simulink model "ex3"  (R2020a)
settings: Solver=VariableStepAuto  StartTime=0.0  StopTime=10.0  RelTol=1e-3
settings Model: Creator=EREN  LastModifiedBy=EREN

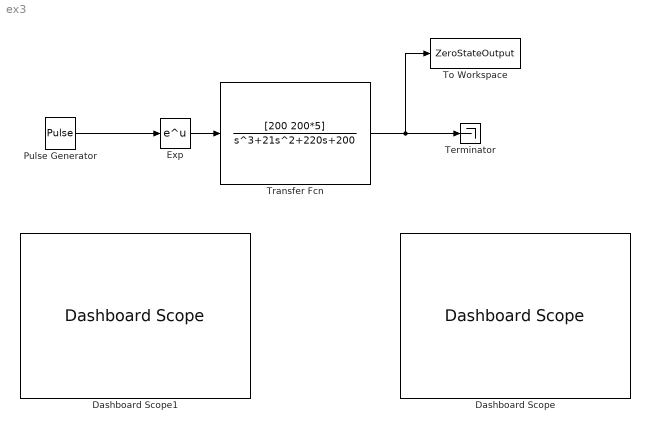
== system ex3 ==
  Dashboard Scope : DashboardScope
  Dashboard Scope1 : DashboardScope
  Exp : Math  SaturateOnIntegerOverflow=on
  Pulse Generator : DiscretePulseGenerator  PulseType=Time based  Amplitude=100  Period=10
  Terminator : Terminator
  To Workspace : ToWorkspace  VariableName=ZeroStateOutput  SaveFormat=Timeseries  SampleTime=-1
  Transfer Fcn : TransferFcn  Numerator=[200 200*5]  Denominator=[1 21 220 200]
  wires:
  Pulse Generator/1 -> Exp/1
  Exp/1 -> Transfer Fcn/1
  Transfer Fcn/1 -> To Workspace/1, Terminator/1
